simulink model "td3"  (Simulink 8.3)
settings: Solver=ode45  StartTime=0.0  StopTime=10.0  RelTol=1e-3
undefined symbols (not defined in the file or in its folder): Nb
libraries: simulink x3
settings Model: Creator=elkhadiy  LastModifiedBy=elkhadiy
settings DataIOCC: SignalLoggingSaveFormat=Dataset
settings DebuggingCC: UnderspecifiedInitializationDetection=Simplified  StateNameClashWarn=none
settings GRTTargetCC: CombineOutputUpdateFcns=on  GRTInterface=off

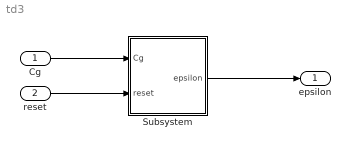
== system td3 ==
  Cg : Inport  OutDataTypeStr=uint32
  reset : Inport  Port=2  OutDataTypeStr=boolean
  Subsystem : Subsystem
  epsilon : Outport  OutDataTypeStr=boolean
  wires:
  Cg/1 -> Subsystem/1(Cg)
  reset/1 -> Subsystem/2(reset)
  Subsystem/1(epsilon) -> epsilon/1

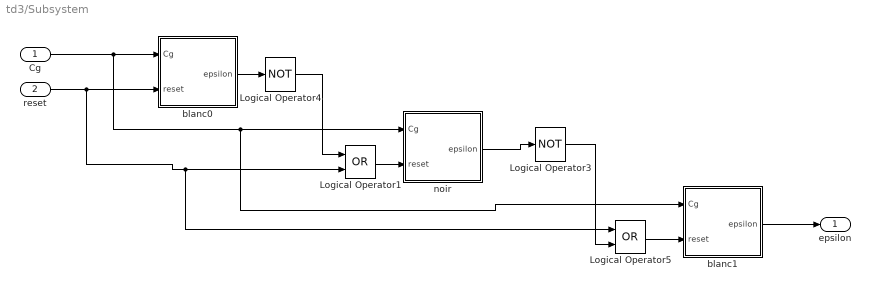
== system td3/Subsystem ==
  Cg : Inport  OutDataTypeStr=uint32
  reset : Inport  Port=2  OutDataTypeStr=boolean
  Logical Operator1 : Logic  Operator=OR  AllPortsSameDT=off  OutDataTypeStr=boolean
  Logical Operator3 : Logic  Operator=NOT  AllPortsSameDT=off  OutDataTypeStr=boolean
  Logical Operator4 : Logic  Operator=NOT  AllPortsSameDT=off  OutDataTypeStr=boolean
  Logical Operator5 : Logic  Operator=OR  AllPortsSameDT=off  OutDataTypeStr=boolean
  blanc0 : Subsystem
  blanc1 : Subsystem
  noir : Subsystem
  epsilon : Outport  OutDataTypeStr=boolean
  wires:
  Cg/1 -> blanc0/1(Cg), blanc1/1(Cg), noir/1(Cg)
  reset/1 -> blanc0/2(reset), Logical Operator5/1, Logical Operator1/2
  blanc1/1(epsilon) -> epsilon/1
  noir/1(epsilon) -> Logical Operator3/1
  Logical Operator1/1 -> noir/2(reset)
  blanc0/1(epsilon) -> Logical Operator4/1
  Logical Operator4/1 -> Logical Operator1/1
  Logical Operator5/1 -> blanc1/2(reset)
  Logical Operator3/1 -> Logical Operator5/2

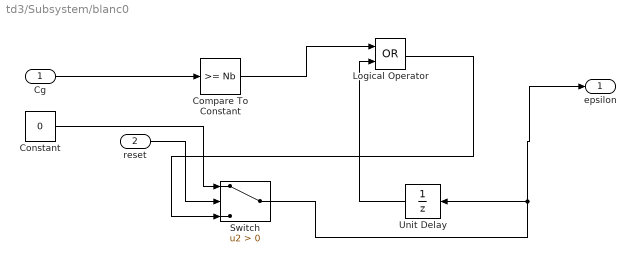
== system td3/Subsystem/blanc0 ==
  Cg : Inport
  reset : Inport  Port=2
  Compare To Constant : simulink/Logic and Bit Operations/Compare To Constant  relop=>=  const=Nb  OutDataTypeStr=boolean
  Constant : Constant  Value=0
  Logical Operator : Logic  Operator=OR  AllPortsSameDT=off  OutDataTypeStr=boolean
  Switch : Switch  Criteria=u2 > Threshold
  Unit Delay : UnitDelay  SampleTime=-1
  epsilon : Outport
  wires:
  Compare To Constant/1 -> Logical Operator/1
  Cg/1 -> Compare To Constant/1
  Logical Operator/1 -> Switch/3
  reset/1 -> Switch/2
  Constant/1 -> Switch/1
  Unit Delay/1 -> Logical Operator/2
  Switch/1 -> epsilon/1, Unit Delay/1

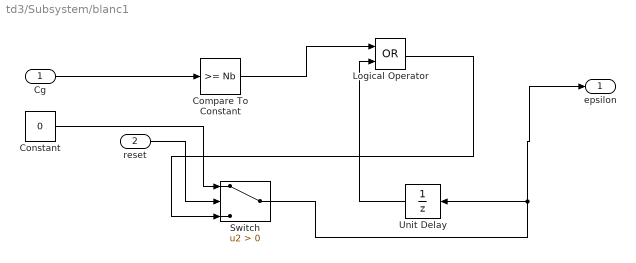
== system td3/Subsystem/blanc1 ==
  Cg : Inport
  reset : Inport  Port=2
  Compare To Constant : simulink/Logic and Bit Operations/Compare To Constant  relop=>=  const=Nb  OutDataTypeStr=boolean
  Constant : Constant  Value=0
  Logical Operator : Logic  Operator=OR  AllPortsSameDT=off  OutDataTypeStr=boolean
  Switch : Switch  Criteria=u2 > Threshold
  Unit Delay : UnitDelay  SampleTime=-1
  epsilon : Outport
  wires:
  Compare To Constant/1 -> Logical Operator/1
  Cg/1 -> Compare To Constant/1
  Logical Operator/1 -> Switch/3
  reset/1 -> Switch/2
  Constant/1 -> Switch/1
  Unit Delay/1 -> Logical Operator/2
  Switch/1 -> epsilon/1, Unit Delay/1

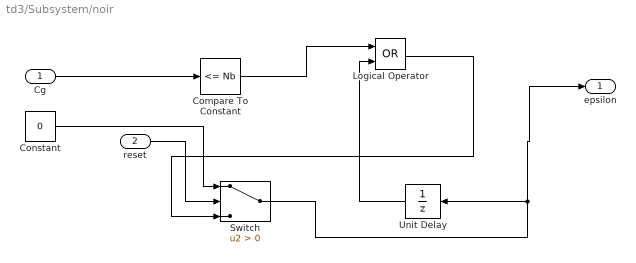
== system td3/Subsystem/noir ==
  Cg : Inport
  reset : Inport  Port=2
  Compare To Constant : simulink/Logic and Bit Operations/Compare To Constant  relop=<=  const=Nb  OutDataTypeStr=boolean
  Constant : Constant  Value=0
  Logical Operator : Logic  Operator=OR  AllPortsSameDT=off  OutDataTypeStr=boolean
  Switch : Switch  Criteria=u2 > Threshold
  Unit Delay : UnitDelay  SampleTime=-1
  epsilon : Outport
  wires:
  Compare To Constant/1 -> Logical Operator/1
  Cg/1 -> Compare To Constant/1
  Logical Operator/1 -> Switch/3
  reset/1 -> Switch/2
  Constant/1 -> Switch/1
  Unit Delay/1 -> Logical Operator/2
  Switch/1 -> epsilon/1, Unit Delay/1
